simulink model "Simulink File"  (R2019a)
settings: Solver=VariableStepAuto  StartTime=0.0  StopTime=30  RelTol=1e-3
values from neighbouring files (symbols this model uses):
  K = acker(A,B,P)    [state_feedback.m]
undefined symbols (not defined in the file or in its folder): A, B, C, D
settings Model: Creator=Sepehr  LastModifiedBy=Sepehr

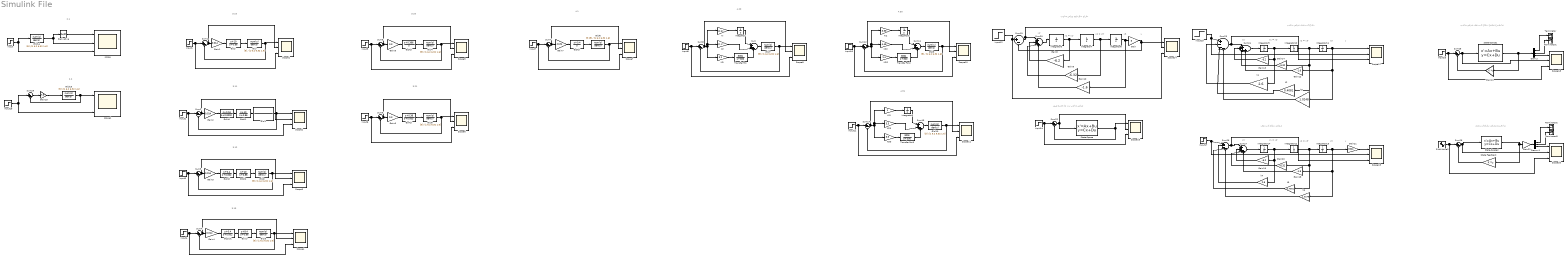
== system Simulink File ==
  note: پیاده سازی معادلات حالت
  note: y
  note: x3
  note: x2 = x3'
  note: x1 = x2'
  note: x1'
  note: x3
  note: y
  note: x1 = x2'
  note: x1'
  note: x2 = x3'
  note: پیاده سازی فیدبک حالت
  note: x2 = x3'
  note: x3
  note: x1'
  note: x1 = x2'
  note: فیدبک حالت نهایی
  note: y
  note: فیدبک حالت نهایی حرفه ای
  note: پیاده سازی فیدبک حالت خیلی حرفه ای
  note: 2.1
  note: 2.2
  note: 3.10
  note: 3.11
  note: 3.12
  note: 3.13
  note: 3.20
  note: 3.21
  note: 4.1
  note: 4.20
  note: 4.30
  note: 4.31
  note: روش حرفه ای تر پیاده سازی
  Demux : Demux  Outputs=3
  Demux1 : Demux  Outputs=3
  Derivative : Derivative
  G(s){,1..5,7,9..10,14..15} (11 alike) : TransferFcn  Numerator=[5]  Denominator=[1 6.2 6.32 1.6]
  G(s)6 : TransferFcn  Numerator=[5 25]  Denominator=[1 6.2 6.32 1.6]
  Gain : Gain  Gain=5
  Gain{1..4} (4 alike) : Gain  Gain=0.014
  Gain10 : Gain  Gain=-1.6
  Gain11 : Gain  Gain=K  Multiplication=Matrix(K*u)
  Gain12 : Gain  Gain=-1.6
  Gain13 : Gain  Gain=-6.2
  Gain14 : Gain  Gain=-6.32
  Gain15 : Gain  Gain=7.5
  Gain18 : Gain  Gain=-1.6
  Gain19 : Gain  Gain=-6.2
  Gain20 : Gain  Gain=-6.32
  Gain21 : Gain  Gain=2.624
  Gain22 : Gain  Gain=2.624
  Gain5 : Gain  Gain=0.3
  Gain6 : Gain  Gain=0.3
  Gain7 : Gain  Gain=0.0656
  Gain8 : Gain  Gain=-6.2
  Gain9 : Gain  Gain=-6.32
  Gc'(s) : TransferFcn  Numerator=[1 8.4]  Denominator=[1 0.86]
  Gc(s) : TransferFcn  Numerator=[1 10]  Denominator=[1 0.86]
  Gc(s)1 : TransferFcn  Numerator=[1 10]  Denominator=[1 0.86]
  Gc(s)2 : TransferFcn  Numerator=[1 10]  Denominator=[1 0.86]
  Gc1(s) : TransferFcn  Numerator=[1 0.04]  Denominator=[1 0.0002]
  Gc2(s) : TransferFcn  Numerator=[1 0.4]  Denominator=[1 0.002]
  Gc2(s)1 : TransferFcn  Numerator=[1 0.4]  Denominator=[1 0.002]
  Gc3(s) : TransferFcn  Numerator=[1 0.366]  Denominator=[1 0]
  Gc4(s) : TransferFcn  Numerator=[1 0.36]  Denominator=[1 0.005]
  Gc5(s) : TransferFcn  Numerator=[1 0.4]  Denominator=[1 0]
  Input{,1..8,10..12,14..17,19} (17 alike) : Step  Time=0  SampleTime=20
  Integrator{,2..3,6..14} (12 alike) : Integrator
  KD : Gain  Gain=3.1
  KD2 : Gain  Gain=1.4
  KD3 : Gain  Gain=3.5
  KI : Gain  Gain=10.61
  KI2 : Gain  Gain=3.58
  KI3 : Gain
  KP : Gain  Gain=11.47
  KP2 : Gain  Gain=4.48
  KP3 : Gain  Gain=3.3
  Scope{1..8,10..11,14,16..20} (16 alike) : Scope  NumInputPorts=3
  Sine Wave2 : Sin  Amplitude=2  SampleTime=0
  State Feedback : Gain  Gain=K  Multiplication=Matrix(K*u)
  State-Space : StateSpace  A=A  B=B  C=C  D=D  InitialCondition=0
  State-Space1 : StateSpace  A=A  B=B  C=eye(3)  D=[0;0;0]  InitialCondition=0
  State-Space2 : StateSpace  A=A  B=B  C=eye(3)  D=[0;0;0]  InitialCondition=0
  Sum : Sum  Inputs=|+++
  Sum{1..8,12,14,19,22,25,28..29} (15 alike) : Sum  Inputs=|+-
  Sum11 : Sum  Inputs=|+++
  Sum13 : Sum  Inputs=|+++
  Sum20 : Sum  Inputs=|++++
  Sum23 : Sum  Inputs=|+---
  Sum24 : Sum  Inputs=|++++
  Sum26 : Sum  Inputs=|+---
  Sum27 : Sum  Inputs=|++++
  Terminator{,1..3} (4 alike) : Terminator
  Transfer Fcn : TransferFcn  Numerator=[300 0]  Denominator=[1 300]
  Transfer Fcn2 : TransferFcn  Numerator=[300 0]  Denominator=[1 300]
  Transfer Fcn3 : TransferFcn  Numerator=[300 0]  Denominator=[1 300]
  k1 : Gain  Gain=2.6
  k2 : Gain  Gain=0.4081
  k3 : Gain  Gain=1.0248
  k4 : Gain  Gain=2.6
  k5 : Gain  Gain=0.4081
  k6 : Gain  Gain=1.0248
  scope : Scope  NumInputPorts=3
  scope1 : Scope  NumInputPorts=3
  wires:
  Input1/1 -> Scope1/3, Sum1/1  "Input"
  G(s)/1 -> Scope1/1, Sum1/2  "Step Response"
  Gain1/1 -> Gc(s)/1
  Gc(s)/1 -> G(s)/1
  Sum1/1 -> Scope1/2, Gain1/1  "error"
  G(s)1/1 -> Scope2/1, Sum2/2  "Step Response"
  Input2/1 -> Scope2/3, Sum2/1  "Input"
  Sum2/1 -> Scope2/2, Gain2/1  "error"
  Gc(s)1/1 -> G(s)1/1
  Gain2/1 -> Gc1(s)/1
  Gc1(s)/1 -> Gc(s)1/1
  Gc2(s)/1 -> Gc(s)2/1
  Gc(s)2/1 -> G(s)2/1
  Sum3/1 -> Scope3/2, Gain3/1  "error"
  G(s)2/1 -> Scope3/1, Sum3/2  "Step Response"
  Input3/1 -> Scope3/3, Sum3/1  "Input"
  Gain3/1 -> Gc2(s)/1
  Gain4/1 -> Gc2(s)1/1
  Input4/1 -> Scope4/3, Sum4/1  "Input"
  Sum4/1 -> Scope4/2, Gain4/1  "error"
  Gc'(s)/1 -> G(s)3/1
  G(s)3/1 -> Scope4/1, Sum4/2  "Step Response"
  Gc2(s)1/1 -> Gc'(s)/1
  Gain5/1 -> Gc3(s)/1
  G(s)4/1 -> Scope5/1, Sum5/2  "Step Response"
  Input5/1 -> Scope5/3, Sum5/1  "Input"
  Sum5/1 -> Scope5/2, Gain5/1  "error"
  Gc3(s)/1 -> G(s)4/1
  Sum6/1 -> Scope6/2, Gain6/1  "error"
  Gc4(s)/1 -> G(s)5/1
  Gain6/1 -> Gc4(s)/1
  Input6/1 -> Scope6/3, Sum6/1  "Input"
  G(s)5/1 -> Scope6/1, Sum6/2  "Step Response"
  Sum7/1 -> Scope7/2, Gain7/1  "error"
  Gc5(s)/1 -> G(s)6/1
  Gain7/1 -> Gc5(s)/1
  Input7/1 -> Scope7/3, Sum7/1  "Input"
  G(s)6/1 -> Scope7/1, Sum7/2  "Step Response"
  Input8/1 -> Scope8/3, Sum8/1  "Input"
  G(s)7/1 -> Scope8/1, Sum8/2  "Step Response"
  Sum8/1 -> KI/1, KP/1, KD/1, Scope8/2  "error"
  KI/1 -> Integrator/1
  Sum/1 -> G(s)7/1
  Integrator/1 -> Sum/1
  KP/1 -> Sum/2
  Transfer Fcn/1 -> Sum/3
  KD/1 -> Transfer Fcn/1
  KD2/1 -> Transfer Fcn2/1
  Transfer Fcn2/1 -> Sum11/3
  KP2/1 -> Sum11/2
  Integrator2/1 -> Sum11/1
  KI2/1 -> Integrator2/1
  Sum11/1 -> G(s)9/1
  Sum12/1 -> KI2/1, KP2/1, KD2/1, Scope10/2  "error"
  G(s)9/1 -> Scope10/1, Sum12/2  "Step Response"
  Input10/1 -> Scope10/3, Sum12/1  "Input"
  Input11/1 -> Scope11/3, Sum14/1  "Input"
  G(s)10/1 -> Scope11/1, Sum14/2  "Step Response"
  Sum14/1 -> KI3/1, KP3/1, KD3/1, Scope11/2  "error"
  Transfer Fcn3/1 -> Sum13/3
  KD3/1 -> Transfer Fcn3/1
  KI3/1 -> Integrator3/1
  Integrator3/1 -> Sum13/1
  KP3/1 -> Sum13/2
  Sum13/1 -> G(s)10/1
  Sum20/1 -> Integrator6/1
  Integrator8/1 -> Gain10/1, Gain/1
  Integrator7/1 -> Gain9/1, Integrator8/1
  Integrator6/1 -> Gain8/1, Integrator7/1
  Gain8/1 -> Sum20/2
  Gain9/1 -> Sum20/3
  Gain10/1 -> Sum20/4
  Gain/1 -> Scope14/1, Sum19/2  "step response"
  Sum19/1 -> Sum20/1, Scope14/2  "error"
  Input12/1 -> Scope14/3, Sum19/1  "Input"
  State-Space/1 -> Scope16/1, Sum22/2  "Step Response"
  Input14/1 -> Scope16/3, Sum22/1  "Input"
  Sum22/1 -> State-Space/1, Scope16/2  "error"
  Input15/1 -> Scope17/2, Sum23/1  "Input"
  Sum23/1 -> Sum24/1, Scope17/3  "error"
  Integrator10/1 -> k2/1, Gain14/1, Integrator11/1
  Sum24/1 -> Integrator9/1
  Gain13/1 -> Sum24/2
  Integrator9/1 -> k1/1, Gain13/1, Integrator10/1
  Gain12/1 -> Sum24/4
  Gain14/1 -> Sum24/3
  k1/1 -> Sum23/2
  k2/1 -> Sum23/3
  k3/1 -> Sum23/4
  State-Space1/1 -> Gain11/1, Demux/1  "Step Response"
  Sum25/1 -> State-Space1/1, Scope18/2  "error"
  Input16/1 -> Scope18/3, Sum25/1  "Input"
  Gain11/1 -> Sum25/2
  Demux/3 -> Scope18/1
  Demux/1 -> Terminator/1
  Demux/2 -> Terminator1/1
  State-Space2/1 -> Gain22/1, State Feedback/1
  k6/1 -> Sum26/4
  Gain18/1 -> Sum27/4
  Gain20/1 -> Sum27/3
  Sum28/1 -> State-Space2/1, Scope20/2  "error"
  Integrator14/1 -> k4/1, Gain19/1, Integrator12/1
  Gain19/1 -> Sum27/2
  Sum27/1 -> Integrator14/1
  Integrator12/1 -> Gain20/1, k5/1, Integrator13/1
  Input17/1 -> Scope19/2, Sum26/1  "Input"
  Demux1/1 -> Terminator2/1
  Sum26/1 -> Scope19/3, Sum27/1  "error"
  Gain21/1 -> Scope19/1
  State Feedback/1 -> Sum28/2
  Integrator13/1 -> Gain18/1, k6/1, Gain21/1  "step response"
  Gain22/1 -> Demux1/1
  k5/1 -> Sum26/3
  Demux1/2 -> Terminator3/1
  Sine Wave2/1 -> Scope20/3, Sum28/1  "Input"
  k4/1 -> Sum26/2
  Demux1/3 -> Scope20/1
  G(s)14/1 -> scope/2, Derivative/1  "Step Response"
  Derivative/1 -> scope/1  "Impact Response"
  Input/1 -> scope/3, G(s)14/1  "Input"
  Input19/1 -> Sum29/1, scope1/3  "Input"
  G(s)15/1 -> scope1/1, Sum29/2
  Gain15/1 -> G(s)15/1
  Sum29/1 -> Gain15/1
  Integrator11/1 -> Scope17/1, k3/1, Gain12/1  "step response"
